simulink model "my_demo2"  (R2012b)
settings: Solver=FixedStepDiscrete  StartTime=0.0  StopTime=Inf  FixedStep=0.033  RelTol=1e-3
values from neighbouring files (symbols this model uses):
  xr = 0    [param.m]
  yr = 0    [param.m]
undefined symbols (not defined in the file or in its folder): magnitude
libraries: simiam x5, simulink x1, vrlib x1
settings Model: Creator=jdelacroix  LastModifiedBy=samati
settings DataIOCC: SignalLoggingSaveFormat=ModelDataLogs  SaveOutput=off  SignalLogging=off  DSMLogging=off  SaveTime=off
settings DebuggingCC: MultiTaskDSMMsg=warning  MultiTaskCondExecSysMsg=none  FcnCallInpInsideContextMsg=EnableAllAsWarning  StrictBusMsg=None
settings RTWCC: IncludeERTFirstTime=on
settings CodeAppCC: CustomSymbolStrType=$N$R$M_T  InternalIdentifier=Shortened
settings GRTTargetCC: CodeReplacementLibrary=None  CPPClassGenCompliant=on

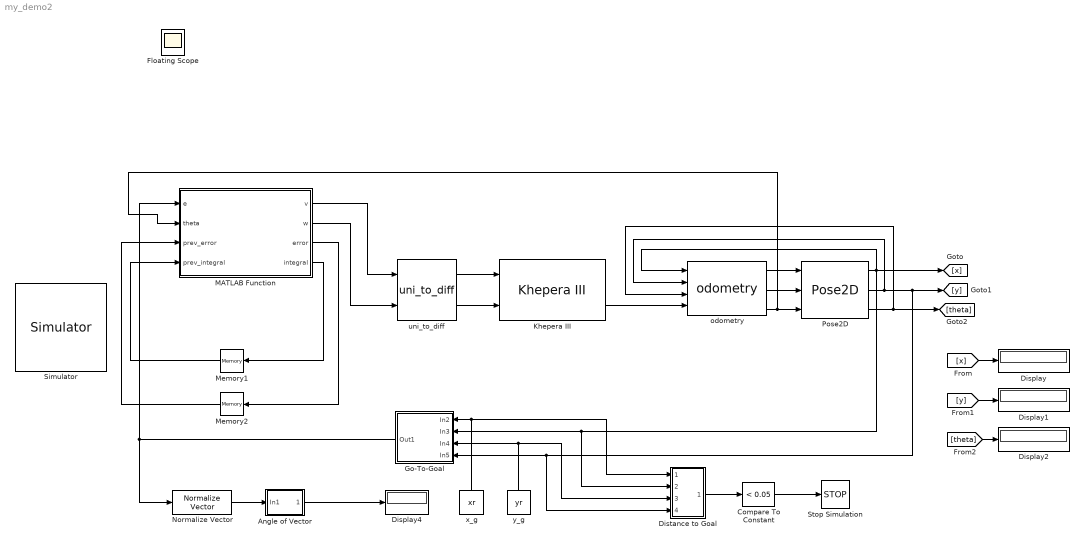
== system my_demo2 ==
  Angle of Vector : Subsystem
      mask Display:
      | port_label('input', 1, 'u')
      | port_label('output', 1, 'theta')
  Compare To Constant : simulink/Logic and Bit Operations/Compare To Constant  relop=<  const=0.05  OutDataTypeStr=boolean
  Display{,1..2,4} (4 alike) : Display
  Distance to Goal : Subsystem
      mask Display:
      | port_label('input', 1, 'x_g')
      | port_label('input', 2, 'x')
      | port_label('input', 3, 'y_g')
      | port_label('input', 4, 'y')
      | port_label('output', 1, 'd')
  Go-To-Goal : Subsystem
      mask Display:
      | port_label('input', 1, 'x_g')
      | port_label('input', 2, 'x')
      | port_label('input', 3, 'y_g')
      | port_label('input', 4, 'y')
      | port_label('output', 1, 'u_gtg')
  Khepera III : simiam/Khepera III  x_0=xi  y_0=yi  theta_0=thetai  robot_id=1
  MATLAB Function : MATLAB Function  TreatAsAtomicUnit=on
  Memory1 : Memory  InheritSampleTime=on  StateIdentifier=state_estimate_theta
  Memory2 : Memory  InheritSampleTime=on  StateIdentifier=state_estimate_theta
  Normalize Vector : vrlib/Utilities/Normalize Vector  maxzero=0
  Pose2D : simiam/Pose2D  SystemSampleTime=-1
  Simulator : simiam/Simulator  Priority=1
  Stop Simulation : Stop
  odometry : simiam/odometry  wheel_radius=r  wheel_base_length=l  ticks_per_rev=ticks
  uni_to_diff : simiam/uni_to_diff  wheel_radius=r  wheel_base_length=l
  x_g : Constant  Value=xr
  y_g : Constant  Value=yr
  Floating Scope : Scope
  wires:
  uni_to_diff/1 -> Khepera III/1
  uni_to_diff/2 -> Khepera III/2
  odometry/3 -> MATLAB Function/2(theta), Pose2D/3
  odometry/2 -> Pose2D/2
  odometry/1 -> Pose2D/1
  Khepera III/2 -> odometry/4
  Pose2D/1 -> [x], odometry/1, Distance to Goal/2(In2), Go-To-Goal/2(In3)
  Pose2D/2 -> [y], Distance to Goal/4(In4), Go-To-Goal/4(In5), odometry/2
  x_g/1 -> Distance to Goal/1(In1), Go-To-Goal/1(In2)
  y_g/1 -> Distance to Goal/3(In3), Go-To-Goal/3(In4)
  Go-To-Goal/1(Out1) -> MATLAB Function/1(e), Normalize Vector/1
  Pose2D/3 -> [theta], odometry/3
  Normalize Vector/1 -> Angle of Vector/1(In1)
  Angle of Vector/1(Out1) -> Display4/1
  Distance to Goal/1(Out1) -> Compare To Constant/1
  Compare To Constant/1 -> Stop Simulation/1
  MATLAB Function/2(w) -> uni_to_diff/2
  MATLAB Function/3(error) -> Memory2/1
  Memory2/1 -> MATLAB Function/3(prev_error)
  MATLAB Function/1(v) -> uni_to_diff/1
  Memory1/1 -> MATLAB Function/4(prev_integral)
  MATLAB Function/4(integral) -> Memory1/1
  [theta] -> Display2/1
  [y] -> Display1/1
  [x] -> Display/1

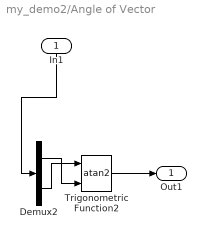
== system my_demo2/Angle of Vector ==
  In1 : Inport
  Demux2 : Demux  Outputs=2
  Trigonometric Function2 : Trigonometry  Operator=atan2
  Out1 : Outport
  wires:
  Trigonometric Function2/1 -> Out1/1
  Demux2/1 -> Trigonometric Function2/2
  Demux2/2 -> Trigonometric Function2/1
  In1/1 -> Demux2/1

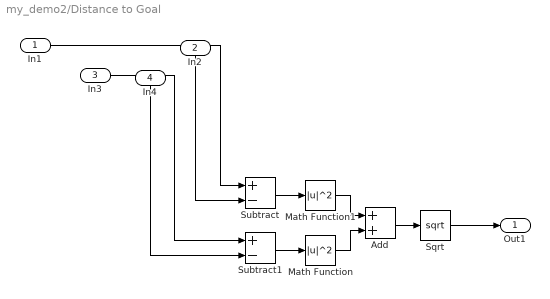
== system my_demo2/Distance to Goal ==
  In1 : Inport
  In2 : Inport  Port=2
  In3 : Inport  Port=3
  In4 : Inport  Port=4
  Add : Sum
  Math Function : Math  Operator=magnitude^2  SaturateOnIntegerOverflow=on
  Math Function1 : Math  Operator=magnitude^2  SaturateOnIntegerOverflow=on
  Sqrt : Sqrt  SaturateOnIntegerOverflow=on
  Subtract : Sum  Inputs=+-
  Subtract1 : Sum  Inputs=+-
  Out1 : Outport
  wires:
  In4/1 -> Subtract1/2
  Subtract1/1 -> Math Function/1
  Math Function/1 -> Add/2
  Sqrt/1 -> Out1/1
  Subtract/1 -> Math Function1/1
  Math Function1/1 -> Add/1
  Add/1 -> Sqrt/1
  In2/1 -> Subtract/2
  In3/1 -> Subtract1/1
  In1/1 -> Subtract/1

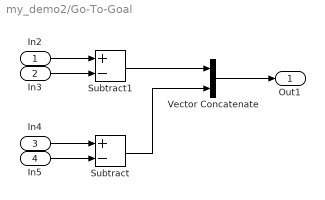
== system my_demo2/Go-To-Goal ==
  In2 : Inport
  In3 : Inport  Port=2
  In4 : Inport  Port=3
  In5 : Inport  Port=4
  Subtract : Sum  Inputs=+-
  Subtract1 : Sum  Inputs=+-
  Vector Concatenate : Concatenate  Mode=Multidimensional array
  Out1 : Outport
  wires:
  In5/1 -> Subtract/2
  In2/1 -> Subtract1/1
  In3/1 -> Subtract1/2
  In4/1 -> Subtract/1
  Vector Concatenate/1 -> Out1/1
  Subtract1/1 -> Vector Concatenate/1
  Subtract/1 -> Vector Concatenate/2

== matlab function my_demo2/MATLAB Function ==
  data: e input; v output; theta input; prev_error input; prev_integral input; w output; error output; integral output
function [v, w, error, integral] = my_demo2(e, theta, prev_error, prev_integral)

u_max = 0.1;
a = 0.1;
k1 = 1./exp(abs(e(1))) + (u_max * (1-exp(-a.*e(1).^2))) ./ abs(e(1));
k2 = 1./exp(abs(e(2))) + (u_max * (1-exp(-a.*e(2).^2))) ./ abs(e(2));

u1 = k1*e(1);
u2 = k2*e(2);

v = sqrt(u1^2 + u2^2);
theta_d = atan2(u2, u1);

Kp = 20;
Ki = 1;
Kd = 0;
dt = 0.033;

error = theta_d - theta;
integral = prev_integral + error*dt;
derivative = (error - prev_error)/dt;
w = Kp*error + Ki*integral + Kd*derivative;
